simulink model "energy_model"  (R2019b)
settings: Solver=VariableStepAuto  StartTime=0.0  StopTime=out.motor1_reference.time(end)  RelTol=1e-3
values from neighbouring files (symbols this model uses):
  c_m = 0.0514    [model_parameters.m]
undefined symbols (not defined in the file or in its folder): J, J_r, M, m
libraries: simulink x3
settings Model: Creator=Олег  LastModifiedBy=Олег
settings DataIOCC: ExternalInput=out

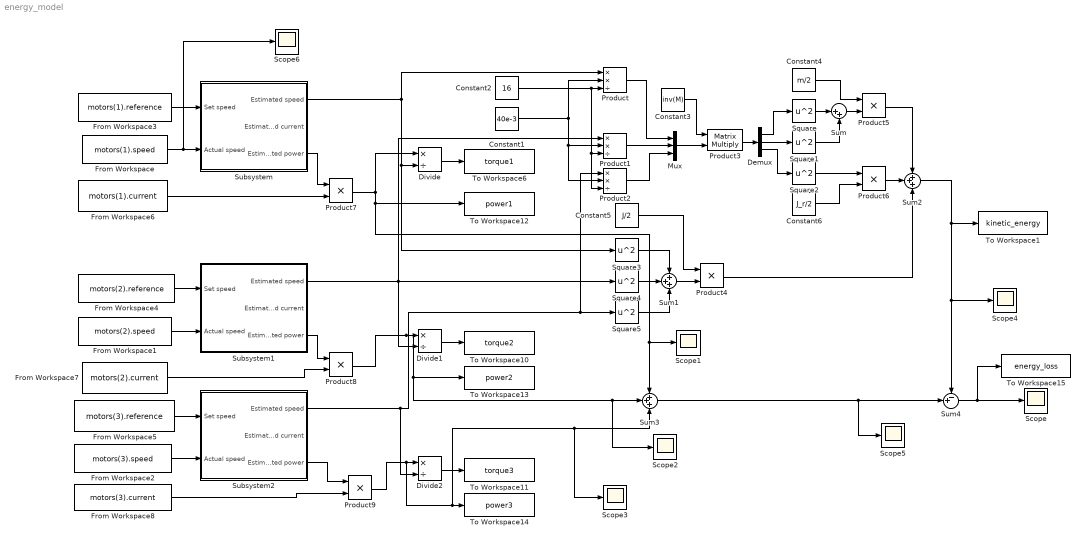
== system energy_model ==
  Constant1 : Constant  Value=40e-3
  Constant2 : Constant  Value=16
  Constant3 : Constant  Value=inv(M)
  Constant4 : Constant  Value=m/2
  Constant5 : Constant  Value=J/2
  Constant6 : Constant  Value=J_r/2
  Demux : Demux  Outputs=3
  Divide : Product  Inputs=*/
  Divide1 : Product  Inputs=*/
  Divide2 : Product  Inputs=*/
  From Workspace : FromWorkspace  VariableName=motors(1).speed  SampleTime=0
  From Workspace1 : FromWorkspace  VariableName=motors(2).speed  SampleTime=0
  From Workspace2 : FromWorkspace  VariableName=motors(3).speed  SampleTime=0
  From Workspace3 : FromWorkspace  VariableName=motors(1).reference  SampleTime=0
  From Workspace4 : FromWorkspace  VariableName=motors(2).reference  SampleTime=0
  From Workspace5 : FromWorkspace  VariableName=motors(3).reference  SampleTime=0
  From Workspace6 : FromWorkspace  VariableName=motors(1).current  SampleTime=0
  From Workspace7 : FromWorkspace  VariableName=motors(2).current  SampleTime=0
  From Workspace8 : FromWorkspace  VariableName=motors(3).current  SampleTime=0
  Mux : Mux  Inputs=3
  Product : Product  Inputs=**/
  Product1 : Product  Inputs=**/
  Product2 : Product  Inputs=**/
  Product3 : Product  Multiplication=Matrix(*)
  Product{4..9} (6 alike) : Product
  Scope{,1..6} (7 alike) : Scope
  Square{,1..5} (6 alike) : Math  Operator=square  SignedPower=off  SaturateOnIntegerOverflow=on
  Subsystem : Subsystem
  Subsystem1 : Subsystem
  Subsystem2 : Subsystem
  Sum : Sum  Inputs=|++
  Sum1 : Sum  Inputs=+++
  Sum2 : Sum  Inputs=+++
  Sum3 : Sum  Inputs=+++
  Sum4 : Sum  Inputs=-+|
  To Workspace1 : ToWorkspace  VariableName=kinetic_energy  SaveFormat=Timeseries  SampleTime=-1
  To Workspace10 : ToWorkspace  VariableName=torque2  SaveFormat=Timeseries  SampleTime=-1
  To Workspace11 : ToWorkspace  VariableName=torque3  SaveFormat=Timeseries  SampleTime=-1
  To Workspace12 : ToWorkspace  VariableName=power1  SaveFormat=Timeseries  SampleTime=-1
  To Workspace13 : ToWorkspace  VariableName=power2  SaveFormat=Timeseries  SampleTime=-1
  To Workspace14 : ToWorkspace  VariableName=power3  SaveFormat=Timeseries  SampleTime=-1
  To Workspace15 : ToWorkspace  VariableName=energy_loss  SaveFormat=Timeseries  SampleTime=-1
  To Workspace6 : ToWorkspace  VariableName=torque1  SaveFormat=Timeseries  SampleTime=-1
  wires:
  From Workspace4/1 -> Subsystem1/1(Set speed)
  From Workspace1/1 -> Subsystem1/2(Actual speed)
  Subsystem1/1(Estimated speed) -> Product1/1, Square4/1, Divide1/2
  Subsystem2/1(Estimated speed) -> Square5/1, Product2/1, Divide2/2
  From Workspace5/1 -> Subsystem2/1(Set speed)
  Square3/1 -> Sum1/1
  Constant4/1 -> Product5/1
  Subsystem/1(Estimated speed) -> Square3/1, Divide/2, Product/1
  Product2/1 -> Mux/3
  From Workspace2/1 -> Subsystem2/2(Actual speed)
  Product3/1 -> Demux/1
  Product1/1 -> Mux/2
  Square/1 -> Sum/1
  Constant2/1 -> Product2/3, Product1/3, Product/3
  Product6/1 -> Sum2/2
  Divide1/1 -> To Workspace10/1
  Square1/1 -> Sum/2
  Divide/1 -> To Workspace6/1
  Sum/1 -> Product5/2
  Constant1/1 -> Product/2, Product1/2, Product2/2
  Square2/1 -> Product6/1
  Product5/1 -> Sum2/1
  Sum4/1 -> Scope/1, To Workspace15/1
  Square4/1 -> Sum1/2
  Divide2/1 -> To Workspace11/1
  Constant5/1 -> Product4/1
  Demux/2 -> Square1/1
  Sum2/1 -> To Workspace1/1, Scope4/1, Sum4/1
  Demux/1 -> Square/1
  Demux/3 -> Square2/1
  From Workspace/1 -> Scope6/1, Subsystem/2(Actual speed)
  From Workspace3/1 -> Subsystem/1(Set speed)
  Square5/1 -> Sum1/3
  Sum1/1 -> Product4/2
  Constant6/1 -> Product6/2
  Sum3/1 -> Scope5/1, Sum4/2
  Product4/1 -> Sum2/3
  Constant3/1 -> Product3/1
  Mux/1 -> Product3/2
  Product/1 -> Mux/1
  From Workspace6/1 -> Product7/2
  Subsystem/3(Estimated power) -> Product7/1
  Product7/1 -> Sum3/1, Scope1/1, To Workspace12/1, Divide/1
  From Workspace7/1 -> Product8/2
  Subsystem1/3(Estimated power) -> Product8/1
  Product8/1 -> To Workspace13/1, Scope2/1, Sum3/2, Divide1/1
  From Workspace8/1 -> Product9/2
  Subsystem2/3(Estimated power) -> Product9/1
  Product9/1 -> Scope3/1, Sum3/3, To Workspace14/1, Divide2/1

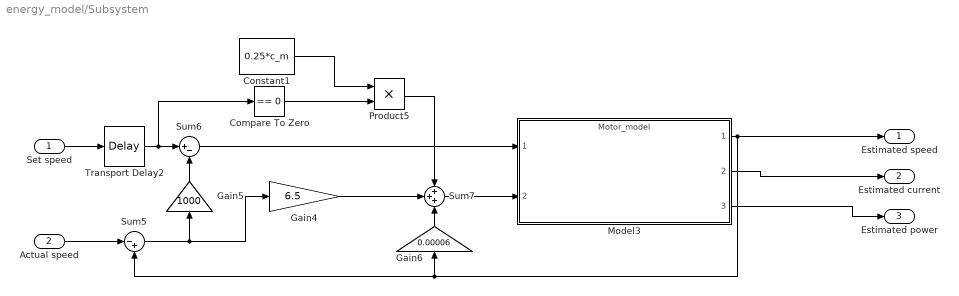
== system energy_model/Subsystem ==
  Set speed : Inport
  Actual speed : Inport  Port=2
  Compare To Zero : simulink/Logic and Bit Operations/Compare To Zero  relop===  OutDataTypeStr=uint8
  Constant1 : Constant  Value=0.25*c_m
  Gain4 : Gain  Gain=6.5
  Gain5 : Gain  Gain=1000
  Gain6 : Gain  Gain=0.00006
  Model3 : ModelReference  ModelNameDialog=Motor_model.slx  SimulationMode=Normal  ModelReferenceVersion=1.133
  Product5 : Product
  Sum5 : Sum  Inputs=|-+
  Sum6 : Sum  Inputs=|+-
  Sum7 : Sum  Inputs=+++
  Transport Delay2 : TransportDelay  DelayTime=0.15
  Estimated speed : Outport
  Estimated current : Outport  Port=2
  Estimated power : Outport  Port=3
  wires:
  Gain6/1 -> Sum7/3
  Gain4/1 -> Sum7/2
  Compare To Zero/1 -> Product5/2
  Sum5/1 -> Gain4/1, Gain5/1
  Sum7/1 -> Model3/2
  Sum6/1 -> Model3/1
  Constant1/1 -> Product5/1
  Transport Delay2/1 -> Sum6/1, Compare To Zero/1
  Set speed/1 -> Transport Delay2/1
  Product5/1 -> Sum7/1
  Actual speed/1 -> Sum5/1
  Gain5/1 -> Sum6/2
  Model3/3 -> Estimated power/1
  Model3/1 -> Estimated speed/1, Sum5/2, Gain6/1
  Model3/2 -> Estimated current/1

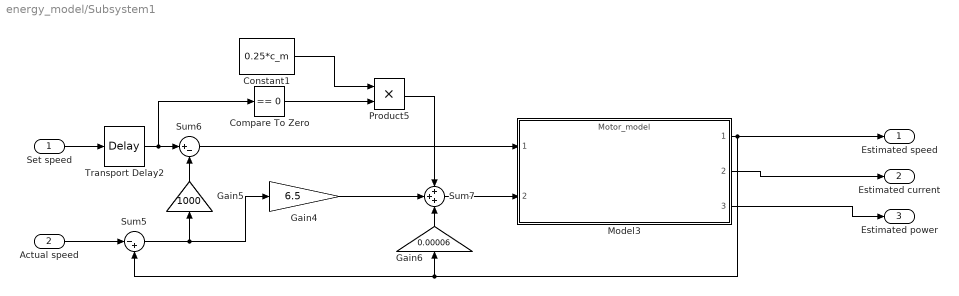
== system energy_model/Subsystem1 ==
  Set speed : Inport
  Actual speed : Inport  Port=2
  Compare To Zero : simulink/Logic and Bit Operations/Compare To Zero  relop===  OutDataTypeStr=uint8
  Constant1 : Constant  Value=0.25*c_m
  Gain4 : Gain  Gain=6.5
  Gain5 : Gain  Gain=1000
  Gain6 : Gain  Gain=0.00006
  Model3 : ModelReference  ModelNameDialog=Motor_model.slx  SimulationMode=Normal  ModelReferenceVersion=1.133
  Product5 : Product
  Sum5 : Sum  Inputs=|-+
  Sum6 : Sum  Inputs=|+-
  Sum7 : Sum  Inputs=+++
  Transport Delay2 : TransportDelay  DelayTime=0.15
  Estimated speed : Outport
  Estimated current : Outport  Port=2
  Estimated power : Outport  Port=3
  wires:
  Gain6/1 -> Sum7/3
  Gain4/1 -> Sum7/2
  Compare To Zero/1 -> Product5/2
  Sum5/1 -> Gain4/1, Gain5/1
  Sum7/1 -> Model3/2
  Sum6/1 -> Model3/1
  Constant1/1 -> Product5/1
  Transport Delay2/1 -> Sum6/1, Compare To Zero/1
  Set speed/1 -> Transport Delay2/1
  Product5/1 -> Sum7/1
  Actual speed/1 -> Sum5/1
  Gain5/1 -> Sum6/2
  Model3/3 -> Estimated power/1
  Model3/1 -> Estimated speed/1, Sum5/2, Gain6/1
  Model3/2 -> Estimated current/1

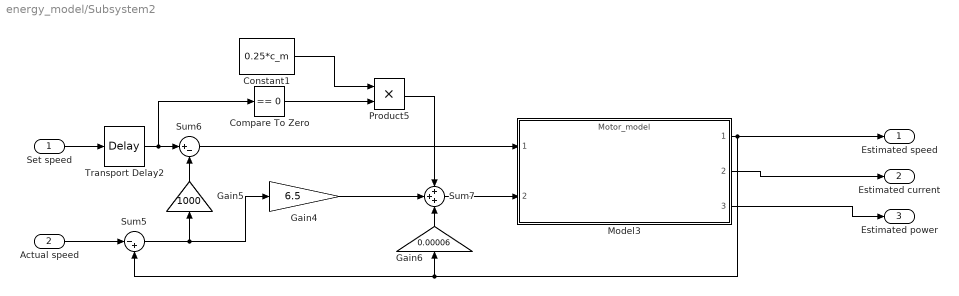
== system energy_model/Subsystem2 ==
  Set speed : Inport
  Actual speed : Inport  Port=2
  Compare To Zero : simulink/Logic and Bit Operations/Compare To Zero  relop===  OutDataTypeStr=uint8
  Constant1 : Constant  Value=0.25*c_m
  Gain4 : Gain  Gain=6.5
  Gain5 : Gain  Gain=1000
  Gain6 : Gain  Gain=0.00006
  Model3 : ModelReference  ModelNameDialog=Motor_model.slx  SimulationMode=Normal  ModelReferenceVersion=1.133
  Product5 : Product
  Sum5 : Sum  Inputs=|-+
  Sum6 : Sum  Inputs=|+-
  Sum7 : Sum  Inputs=+++
  Transport Delay2 : TransportDelay  DelayTime=0.15
  Estimated speed : Outport
  Estimated current : Outport  Port=2
  Estimated power : Outport  Port=3
  wires:
  Gain6/1 -> Sum7/3
  Gain4/1 -> Sum7/2
  Compare To Zero/1 -> Product5/2
  Sum5/1 -> Gain4/1, Gain5/1
  Sum7/1 -> Model3/2
  Sum6/1 -> Model3/1
  Constant1/1 -> Product5/1
  Transport Delay2/1 -> Sum6/1, Compare To Zero/1
  Set speed/1 -> Transport Delay2/1
  Product5/1 -> Sum7/1
  Actual speed/1 -> Sum5/1
  Gain5/1 -> Sum6/2
  Model3/3 -> Estimated power/1
  Model3/1 -> Estimated speed/1, Sum5/2, Gain6/1
  Model3/2 -> Estimated current/1
